simulink model "Lab_Modulation_AM"  (R2021b)
settings: Solver=VariableStepAuto  StartTime=0.0  StopTime=10.0  RelTol=1e-3
libraries: dspfdesign x1
settings Model: Creator=User  LastModifiedBy=aleksejshevcenko
settings SolverCC: AlgebraicLoopSolver=TrustRegion
settings DataIOCC: ReturnWorkspaceOutputs=off
settings DebuggingCC: SFMachineParentedDataDiag=warning  ArithmeticOperatorsInVariantConditions=warning
settings SFSimCC: SimUseLocalCustomCode=off  CustomCodeUndefinedFunction=UseInterfaceOnly
settings RTWCC: RTWUseLocalCustomCode=off
settings CodeAppCC: StateflowObjectComments=on

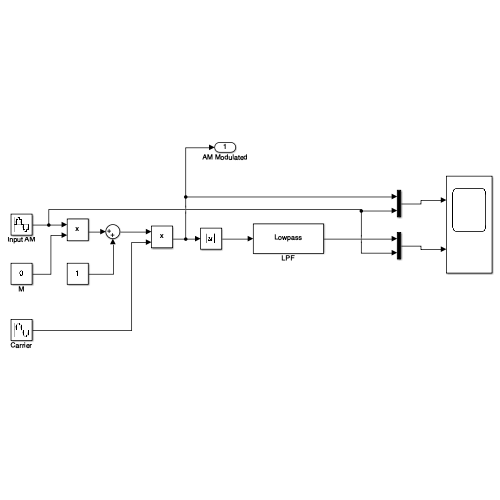
[thumbnail: Simulink's stored preview of the top-level diagram]
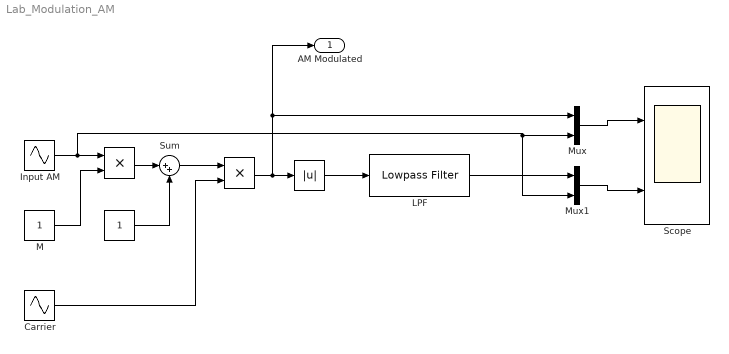
== system Lab_Modulation_AM ==
  " " : Constant
  " " : Product
  " " : Product
  " " : Abs
  "Carrier " : Sin  Frequency=100*2*pi  SampleTime=0.0001
  "Input AM " : Sin  Frequency=2*2*pi  SampleTime=0.0001
  "LPF " : dspfdesign/Lowpass Filter  FilterType=FIR  DesignForMinimumOrder=on  FilterOrder=50  PassbandFrequency=0.1  StopbandFrequency=100  PassbandRipple=0.1  StopbandAttenuation=80  InheritSampleRate=on  SampleRate=44100  SimulateUsing=Interpreted execution  roundingMode=Floor  coeffsDataTypeStr=fixdt(1,16)
  M : Constant
  Mux : Mux  Inputs=2
  Mux1 : Mux  Inputs=2
  Scope : Scope  NumInputPorts=2
  Sum : Sum  Inputs=|++
  AM Modulated : Outport
  wires:
  M/1 -> " "/2
  "Input AM "/1 -> Mux/2, Mux1/2, " "/1
  " "/1 -> Sum/2
  " "/1 -> Sum/1
  Sum/1 -> " "/1
  "Carrier "/1 -> " "/2
  " "/1 -> Mux/1, AM Modulated/1, " "/1
  " "/1 -> "LPF "/1
  "LPF "/1 -> Mux1/1
  Mux/1 -> Scope/1
  Mux1/1 -> Scope/2
